simulink model "I2C_Master_IWDG"  (R2015b)
settings: Solver=FixedStepDiscrete  StartTime=0.0  StopTime=10.0  FixedStep=0.5  RelTol=1e-3
libraries: I2C_Lib x4, WDG_Lib x1, STM32_Config_Lib x1
settings Model: Creator=liprandd  LastModifiedBy=reynaudp
settings DataIOCC: SaveFormat=Array  SignalLoggingSaveFormat=ModelDataLogs
settings OptimizationCC: OptimizeModelRefInitCode=on  LifeSpan=1
settings DebuggingCC: UnderspecifiedInitializationDetection=Classic  MergeDetectMultiDrivingBlocksExec=none  SolverPrmCheckMsg=warning  MultiTaskDSMMsg=warning  MultiTaskCondExecSysMsg=none
settings HardwareCC: ProdBitPerPointer=32  ProdLargestAtomicInteger=Integer  ProdWordSize=32  ProdHWDeviceType=STMicroelectronics->STM32 32-bit Cortex-M
settings RTWCC: SystemTargetFile=stm32.tlc  TemplateMakefile=stm32.tmf  Description=stm32 (Embedded Target)  GenerateReport=on  LaunchReport=on
settings CodeAppCC: IgnoreCustomStorageClasses=off  MaxIdLength=64  CustomSymbolStrType=$N$R$M
settings STFCustomTargetCC: CodeReplacementLibrary=ARM CMSIS SIN COS  ParMdlRefBuildCompliant=on  ConcurrentExecutionCompliant=off  IncludeMdlTerminateFcn=off  GeneratePreprocessorConditionals=Use local settings  CombineOutputUpdateFcns=on  ERTCustomFileBanners=on  SupportContinuousTime=off  SupportNonInlinedSFcns=off  MATLABClassNameForMDSCustomization=Simulink.SoftwareTarget.ERTCustomization  CPPClassGenCompliant=off  GRTInterface=off  SystemTargetFile=stm32.tlc
settings ERTTargetCC: CodeReplacementLibrary=ARM CMSIS SIN COS  CompOptLevelCompliant=off  ConcurrentExecutionCompliant=off  IncludeMdlTerminateFcn=off  ERTFirstTimeCompliant=off  ModelStepFunctionPrototypeControlCompliant=off  CPPClassGenCompliant=off  UseToolchainInfoCompliant=off  ERTSrcFileBannerTemplate=sourceFileTemplate.cgt  ERTHdrFileBannerTemplate=sourceFileTemplate.cgt  ERTDataSrcFileTemplate=sourceFileTemplate.cgt  ERTDataHdrFileTemplate=sourceFileTemplate.cgt  ERTCustomFileTemplate=customRoutineProcess.tlc
settings ConfigComp: CovModelRefEnable=Off  CovSFcnEnable=off

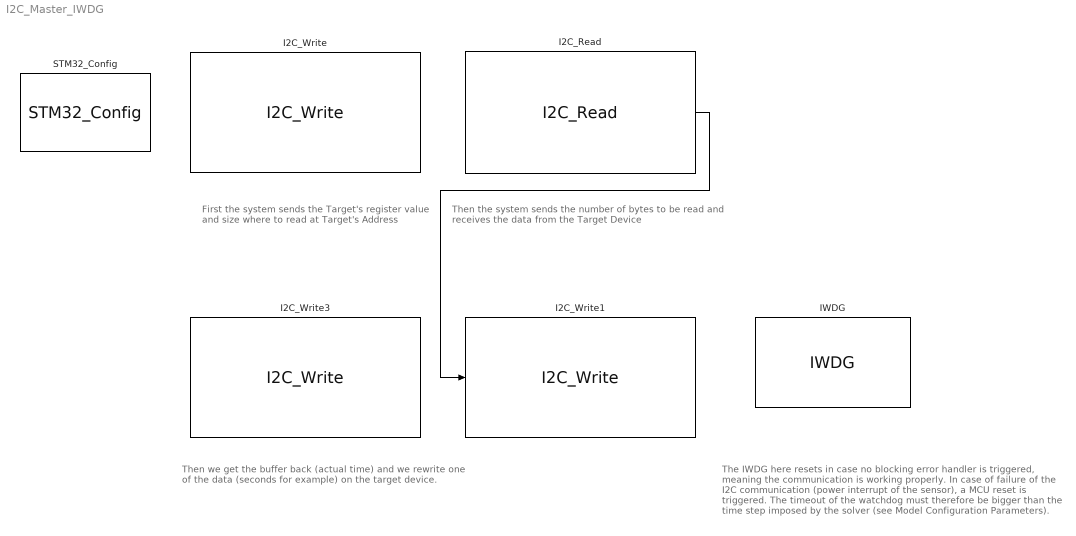
== system I2C_Master_IWDG ==
  note: First the system sends the
      | Target's register value and size
      | where to read at Target's Address
  note: Then the system sends the
      | number of bytes to be read and
      | receives the data from the Target Device
  note: Then we get the buffer back (actual time)
      | and we rewrite one of the data (seconds
      | for example) on the target device.
  note: The IWDG here resets in case no blocking
      | error handler is triggered, meaning the
      | communication is working properly. In case
      | of failure of the I2C communication (power
      | interrupt of the sensor), a MCU reset is triggered.
      | The timeout of the watchdog must therefore be
      | bigger than the time step imposed by the solver
      | (see Model Configuration Parameters).
  I2C_Read : I2C_Lib/I2C_Read  Priority=1  i2cx=I2C1  Device_Mode=MASTER  Device_Address=62  i2c_Mode=DMA_RX_TX  Target_Address=0  handler=hi2c1  Buffer_Size=3  Timeout=50  TimeoutValue=25  Enable_Output=on  Error=off  CallBack=off
  I2C_Write : I2C_Lib/I2C_Write  Priority=0  i2cx=I2C1  Device_Mode=MASTER  Target_Address=160  Target_Register=2  Enable_Input=off  Data_str={2}  i2c_Mode=DMA_RX_TX  Buffer_Size=1  handler=hi2c1  Timeout=50  TimeoutValue=25  Error=off  CallBack=off
  I2C_Write1 : I2C_Lib/I2C_Write  Priority=3  i2cx=I2C1  Device_Mode=MASTER  Target_Address=160  Target_Register=2  Enable_Input=on  Data_str_user=0x02,0x44,0x12  Data_str={2,0x02,0x44,0x12}  i2c_Mode=DMA_RX_TX  Buffer_Size=3  handler=hi2c1  Timeout=50  TimeoutValue=25  Error=off  CallBack=off
  I2C_Write3 : I2C_Lib/I2C_Write  Priority=2  i2cx=I2C1  Device_Mode=MASTER  Target_Address=160  Target_Register=2  Enable_Input=off  Data_str={2}  i2c_Mode=DMA_RX_TX  Buffer_Size=1  handler=hi2c1  Timeout=50  TimeoutValue=25  Error=off  CallBack=off
  IWDG : WDG_Lib/IWDG  Reload=7  Custom_Reload=on  Period=56 ms
  STM32_Config : STM32_Config_Lib/STM32_Config  Project_Path=.\  Config_File=I2C_Master_IWDG.ioc  MCU_Name=STM32F429ZITx
  wires:
  I2C_Read/1 -> I2C_Write1/1
